simulink library "lib_energy_storage2"  (Simulink 4.1.1)
values from neighbouring files (symbols this model uses):
  logFlag = 1    [advSACompMaskInit.m]    (also in advSACompMaskInitR13.m)
undefined symbols (not defined in the file or in its folder): air_cp, amb_tmp, cyc_mph, enable_stop, ess_cap_scale, ess_cb, ess_cc, ess_coulombic_eff, ess_init_soc, ess_max_ah_cap, ess_max_p, ess_max_p_soc, ess_max_soc, ess_max_volts, ess_min_soc, ess_min_volts, ess_MMi, ess_MMo, ess_mod_airflow, ess_mod_cp, ess_mod_cpm, ess_mod_init_tmp, ess_module_mass, ess_module_num, ess_on, ess_parallel_mod_num, ess_res_scale_coef, ess_res_scale_fun, ess_set_tmp, ess_soc, ess_th_calc, ess_th_res, ess_th_res_off, ess_th_res_on, ess_tmp, ess_voc, fund_byu, fund_byuop, mc_min_volts, saber_air_temp, Saber_Battery_IO_File, saber_init_soc, saber_init_temp, saber_init_voc, saber_k_cb, saber_k_cc, saber_k_rc, saber_k_re, saber_k_rt, saber_k_soc, t_soc, time_step
libraries: simulink3 x16, lib_energy_storage x1, lib_energy_storage2 x1
(part 9 of 10)

== system lib_energy_storage2/energy storage <ess> Saber/energy storage <ess> Saber/model/Voltages ==
  Saber Voltages : Inport  Port=1  LatchInput=off
  # batteries : Gain  Gain=ess_module_num  Multiplication=Element-wise(K.*u)  SaturateOnIntegerOverflow=on
  Sum : Sum  Inputs=1  SaturateOnIntegerOverflow=on
  enhancedToWorkspace : Subsystem  TreatAsAtomicUnit=on  mask(enhancedToWorkspace){generalName=generalName, specificName=saber_ess_voltage, logFlag=logFlag}
      mask prompts: generalName "General Name [char-evaluated]"; specificName "Specific Name [char-literal]"; logFlag "Enable flag (1=on,0=off)"
      mask help: A wrapper for the Simulink "To Workspace" block that allows you to evaluate the name of the variable to log to workspace. This is useful to avoid the double logging errors that occur when you pull in two library models that attempt to log to the same variable.
      mask init:
      | enhancedToWsMaker
      settings: CopyFcn=breakLinkCopyFcn  ParentCloseFcn=breakLinkParCloseFcn  RTWFcnNameOpts=Auto  RTWFileNameOpts=Auto
      mask Help:
      | <h2>Enhanced To Workspace Block</h2>
      | <h3>Parameters</h3>
      | <UL>
      | <li><b>General Name:</b> This is the more general name of the variable. Variables are saved to the workspace as <i>generalName_specificName</i>. Note that this is an evaluated variable. If you would like to type in the value directly, it must be surrounded with single quotes. Otherwise you can input the name of a variable containing a char string.</li>
      | <li><b>Specific Name:</b> This is the specific name of the variable. Note that this is input as a char literal (i.e., you don't need quotes).</li>
      | <li><b>Enable Flag:</b> This flag should have the value of 0 or 1. If 0, the variable will not be logged to the workspace. If 1, the variable will be logged. This is done so that variable logging can be turned off to improve speed.</li>
      | </ul>
      | <h3>Overview</h3>
      | <p>The enhanced to workspace block was put together to allow one to dynamically resolve variable names at run time in simulink. This is most powerful when used in conjunction with a masked subsystem to allow multiple instances of that masked subsytem to be used in the same model. The strategy is to set the generalName in the block mask which will allow the block to change the general name for all variable logging on the fly.
      | <h3>Helper Files</h3>
      | <p>Three m-files are required by the enhancedToWorkspace block. These files are located in the &lt; ADVISOR root &gt;/GUI directory :
      | <ul>
      | <li><i>enhancedToWsMaker.m</i> This file runs the mask initialization for the block</li>
      | <li><i>breakLinkCopyFcn.m</i> This file is used by the block callback when the simulink block is copied. It is necessary to break the link to the enhancedToWorkspace similar to the To Workspace block in order for it to be able to configure itself. (Try copying simulink's To Workspace block--it is impossible to make a link)</li>
      | <li><i>breakLinkParCloseFcn.m</i> This file is similar to the breakLinkCopyFcn and is used when a parent system is closed</li>
      | </ul>
      | <hr>
      | 
      | <p>Created 2003-Jan-21, Michael Patrick O'Keefe, NREL</p>
      | 
      | <!--
      | <VARDEF>
      | <H3>var_name</H3>
      | <UL>
      | <LI><B>data type</B> data type here</LI>
      | <LI><B>units</B> units here</LI>
      | <LI><B>vehicle type</B> vehicle type here</LI>
      | <LI><B>description</B> description here</LI>
      | </UL>
      | </VARDEF>
      | -->
      mask Display: disp([generalName,'_',specificName])
  enhancedToWorkspace1 : Subsystem  TreatAsAtomicUnit=on  mask(enhancedToWorkspace){generalName=generalName, specificName=voltage, logFlag=logFlag}
      mask prompts: generalName "General Name [char-evaluated]"; specificName "Specific Name [char-literal]"; logFlag "Enable flag (1=on,0=off)"
      mask help: A wrapper for the Simulink "To Workspace" block that allows you to evaluate the name of the variable to log to workspace. This is useful to avoid the double logging errors that occur when you pull in two library models that attempt to log to the same variable.
      mask init:
      | enhancedToWsMaker
      settings: CopyFcn=breakLinkCopyFcn  ParentCloseFcn=breakLinkParCloseFcn  RTWFcnNameOpts=Auto  RTWFileNameOpts=Auto
      mask Help:
      | <h2>Enhanced To Workspace Block</h2>
      | <h3>Parameters</h3>
      | <UL>
      | <li><b>General Name:</b> This is the more general name of the variable. Variables are saved to the workspace as <i>generalName_specificName</i>. Note that this is an evaluated variable. If you would like to type in the value directly, it must be surrounded with single quotes. Otherwise you can input the name of a variable containing a char string.</li>
      | <li><b>Specific Name:</b> This is the specific name of the variable. Note that this is input as a char literal (i.e., you don't need quotes).</li>
      | <li><b>Enable Flag:</b> This flag should have the value of 0 or 1. If 0, the variable will not be logged to the workspace. If 1, the variable will be logged. This is done so that variable logging can be turned off to improve speed.</li>
      | </ul>
      | <h3>Overview</h3>
      | <p>The enhanced to workspace block was put together to allow one to dynamically resolve variable names at run time in simulink. This is most powerful when used in conjunction with a masked subsystem to allow multiple instances of that masked subsytem to be used in the same model. The strategy is to set the generalName in the block mask which will allow the block to change the general name for all variable logging on the fly.
      | <h3>Helper Files</h3>
      | <p>Three m-files are required by the enhancedToWorkspace block. These files are located in the &lt; ADVISOR root &gt;/GUI directory :
      | <ul>
      | <li><i>enhancedToWsMaker.m</i> This file runs the mask initialization for the block</li>
      | <li><i>breakLinkCopyFcn.m</i> This file is used by the block callback when the simulink block is copied. It is necessary to break the link to the enhancedToWorkspace similar to the To Workspace block in order for it to be able to configure itself. (Try copying simulink's To Workspace block--it is impossible to make a link)</li>
      | <li><i>breakLinkParCloseFcn.m</i> This file is similar to the breakLinkCopyFcn and is used when a parent system is closed</li>
      | </ul>
      | <hr>
      | 
      | <p>Created 2003-Jan-21, Michael Patrick O'Keefe, NREL</p>
      | 
      | <!--
      | <VARDEF>
      | <H3>var_name</H3>
      | <UL>
      | <LI><B>data type</B> data type here</LI>
      | <LI><B>units</B> units here</LI>
      | <LI><B>vehicle type</B> vehicle type here</LI>
      | <LI><B>description</B> description here</LI>
      | </UL>
      | </VARDEF>
      | -->
      mask Display: disp([generalName,'_',specificName])
  ADV Voltage : Outport  Port=1
  tag scope: bus_voltage=scoped
  wires:
  # batteries/1 -> Sum/1, enhancedToWorkspace/1(In1)
  Sum/1 -> [bus_voltage], enhancedToWorkspace1/1(In1), ADV Voltage/1
  Saber Voltages/1 -> # batteries/1

== system lib_energy_storage2/energy storage <ess> Saber/energy storage <ess> Saber/model/enhancedToWorkspace ==
  In1 : Inport  Port=1  LatchInput=off
  Terminator : Terminator
  wires:
  In1/1 -> Terminator/1

== system lib_energy_storage2/energy storage <ess> Saber/energy storage <ess> Saber/model/max pack pwr (W) ==
  note: Edit in the future
      | Used in series power follower
  Ground : Ground
  tag scope: ess_max_pwr=scoped
  wires:
  Ground/1 -> [ess_max_pwr]

== system lib_energy_storage2/energy storage <ess> fundamental model/energy storage <ess> fundamental model/model/Block NOTES ==
  note: Fundamentally based SOC model developed at BYU
      | Files needed:
      | input1.dat
      | input2.dat
      | input3.dat
      | nrel13cs.dll

== system lib_energy_storage2/energy storage <ess> fundamental model/energy storage <ess> fundamental model/model/enhancedToWorkspace ==
  In1 : Inport  Port=1  LatchInput=off
  Terminator : Terminator
  wires:
  In1/1 -> Terminator/1

== system lib_energy_storage2/energy storage <ess> fundamental model/energy storage <ess> fundamental model/model/enhancedToWorkspace1 ==
  In1 : Inport  Port=1  LatchInput=off
  Terminator : Terminator
  wires:
  In1/1 -> Terminator/1

== system lib_energy_storage2/energy storage <ess> fundamental model/energy storage <ess> fundamental model/model/enhancedToWorkspace2 ==
  In1 : Inport  Port=1  LatchInput=off
  Terminator : Terminator
  wires:
  In1/1 -> Terminator/1

== system lib_energy_storage2/energy storage <ess> fundamental model/energy storage <ess> fundamental model/model/enhancedToWorkspace3 ==
  In1 : Inport  Port=1  LatchInput=off
  Terminator : Terminator
  wires:
  In1/1 -> Terminator/1

== system lib_energy_storage2/energy storage <ess> fundamental model/energy storage <ess> fundamental model/model/enhancedToWorkspace4 ==
  In1 : Inport  Port=1  LatchInput=off
  Terminator : Terminator
  wires:
  In1/1 -> Terminator/1

== system lib_energy_storage2/energy storage <ess> fundamental model/energy storage <ess> fundamental model/model/enhancedToWorkspace5 ==
  In1 : Inport  Port=1  LatchInput=off
  Terminator : Terminator
  wires:
  In1/1 -> Terminator/1

== system lib_energy_storage2/energy storage <ess> fundamental model/energy storage <ess> fundamental model/model/enhancedToWorkspace6 ==
  In1 : Inport  Port=1  LatchInput=off
  Terminator : Terminator
  wires:
  In1/1 -> Terminator/1

== system lib_energy_storage2/energy storage <ess> fundamental model/energy storage <ess> fundamental model/model/enhancedToWorkspace7 ==
  In1 : Inport  Port=1  LatchInput=off
  Terminator : Terminator
  wires:
  In1/1 -> Terminator/1

== system lib_energy_storage2/energy storage <ess> fundamental model/energy storage <ess> fundamental model/model/ess tmp ==
  Qess_gen : Inport  Port=1  LatchInput=off
  Enable : EnablePort  StatesWhenEnabling=reset
  #of mods : Gain  Gain=ess_module_num  Multiplication=Element-wise(K.*u)  SaturateOnIntegerOverflow=on
  1/#of mods : Gain  Gain=1/ess_module_num  Multiplication=Element-wise(K.*u)  SaturateOnIntegerOverflow=on
  1/mcp : Gain  Gain=1/(ess_module_mass*ess_mod_cp)  Multiplication=Element-wise(K.*u)  SaturateOnIntegerOverflow=on
  Block NOTES : Subsystem
      settings: RTWFcnNameOpts=Auto  RTWFileNameOpts=Auto
      mask Display: disp('Block\nNOTES')
  Memory : Memory  Orientation=left  X0=cyc_mph(1,2)*.447  InheritSampleTime=off
      settings: RTWStateStorageClass=Auto
  Memory1 : Memory  Orientation=left  X0=cyc_mph(1,2)*.447  InheritSampleTime=off
      settings: RTWStateStorageClass=Auto
  Mux20 : Mux  Inputs=3
      settings: DisplayOption=none
  Qc : Sum  Inputs=++  SaturateOnIntegerOverflow=on
  Qess_case : Fcn  Expr=(u(2) - u(1))/u(3)
  Saturation3 : Saturate  Orientation=left  UpperLimit=1  LowerLimit=0  LinearizeAsGain=on
  Tair,ave : Subsystem  TreatAsAtomicUnit=on
      settings: RTWFcnNameOpts=Auto  RTWFileNameOpts=Auto
  Tess2 : Integrator  ExternalReset=none  InitialConditionSource=internal  InitialCondition=ess_mod_init_tmp  LimitOutput=off  UpperSaturationLimit=inf  LowerSaturationLimit=-inf  ShowSaturationPort=off  ShowStatePort=off  AbsoluteTolerance=auto
  thermostat : Fcn  Orientation=left  Expr=u(1) - ess_set_tmp
  Tess : Outport  Port=1  InitialOutput=0
  Tair : Outport  Port=2
  Qair : Outport  Port=3  OutputWhenDisabled=reset  InitialOutput=0
  wires:
  Tair,ave/1(Tair_ave) -> Tair/1, Mux20/2
  Tair,ave/2(Th Res) -> Mux20/3
  Mux20/1 -> Qess_case/1
  #of mods/1 -> Qair/1
  Memory/1 -> Tair,ave/1(Qess_case)
  Memory1/1 -> Tair,ave/Enable
  Saturation3/1 -> Memory1/1
  thermostat/1 -> Saturation3/1
  1/#of mods/1 -> Qc/2
  Qess_gen/1 -> 1/#of mods/1
  Tess2/1 -> thermostat/1, Mux20/1, Tess/1
  1/mcp/1 -> Tess2/1
  Qess_case/1 -> #of mods/1, Memory/1, Qc/1
  Qc/1 -> 1/mcp/1

== system lib_energy_storage2/energy storage <ess> fundamental model/energy storage <ess> fundamental model/model/max pack pwr (W) ==
  SOC : Inport  Port=1  LatchInput=off
  # batteries : Gain  Gain=ess_module_num  Multiplication=Element-wise(K.*u)  SaturateOnIntegerOverflow=on
  max power : Lookup  InputValues=ess_max_p_soc  OutputValues=ess_max_p
  ess discharge pwr : Outport  Port=1  InitialOutput=0
  wires:
  # batteries/1 -> ess discharge pwr/1
  max power/1 -> # batteries/1
  SOC/1 -> max power/1

== system lib_energy_storage2/energy storage <ess> fundamental model/energy storage <ess> fundamental model/model/stop sim ==
  SOC : Inport  Port=1  LatchInput=off
  Enable : EnablePort
  Const : Constant  Orientation=up  Value=0.1
  Relational Operator : RelationalOperator  Operator=<
  Stop Simulation : Stop
  wires:
  Relational Operator/1 -> Stop Simulation/1
  SOC/1 -> Relational Operator/1
  Const/1 -> Relational Operator/2

== system lib_energy_storage2/energy storage <ess> optima fundamental model/energy storage <ess> optima fundamental model/model/Block NOTES ==
  note: Fundamentally based SOC model developed at BYU
      | Files needed:
      | input1.dat
      | input2.dat
      | input3.dat
      | nrel13cs.dll

== system lib_energy_storage2/energy storage <ess> optima fundamental model/energy storage <ess> optima fundamental model/model/enhancedToWorkspace ==
  In1 : Inport  Port=1  LatchInput=off
  Terminator : Terminator
  wires:
  In1/1 -> Terminator/1

== system lib_energy_storage2/energy storage <ess> optima fundamental model/energy storage <ess> optima fundamental model/model/enhancedToWorkspace1 ==
  In1 : Inport  Port=1  LatchInput=off
  Terminator : Terminator
  wires:
  In1/1 -> Terminator/1

== system lib_energy_storage2/energy storage <ess> optima fundamental model/energy storage <ess> optima fundamental model/model/enhancedToWorkspace2 ==
  In1 : Inport  Port=1  LatchInput=off
  Terminator : Terminator
  wires:
  In1/1 -> Terminator/1

== system lib_energy_storage2/energy storage <ess> optima fundamental model/energy storage <ess> optima fundamental model/model/enhancedToWorkspace3 ==
  In1 : Inport  Port=1  LatchInput=off
  Terminator : Terminator
  wires:
  In1/1 -> Terminator/1

== system lib_energy_storage2/energy storage <ess> optima fundamental model/energy storage <ess> optima fundamental model/model/enhancedToWorkspace4 ==
  In1 : Inport  Port=1  LatchInput=off
  Terminator : Terminator
  wires:
  In1/1 -> Terminator/1

== system lib_energy_storage2/energy storage <ess> optima fundamental model/energy storage <ess> optima fundamental model/model/enhancedToWorkspace5 ==
  In1 : Inport  Port=1  LatchInput=off
  Terminator : Terminator
  wires:
  In1/1 -> Terminator/1

== system lib_energy_storage2/energy storage <ess> optima fundamental model/energy storage <ess> optima fundamental model/model/enhancedToWorkspace6 ==
  In1 : Inport  Port=1  LatchInput=off
  Terminator : Terminator
  wires:
  In1/1 -> Terminator/1

== system lib_energy_storage2/energy storage <ess> optima fundamental model/energy storage <ess> optima fundamental model/model/enhancedToWorkspace7 ==
  In1 : Inport  Port=1  LatchInput=off
  Terminator : Terminator
  wires:
  In1/1 -> Terminator/1

== system lib_energy_storage2/energy storage <ess> optima fundamental model/energy storage <ess> optima fundamental model/model/ess tmp ==
  Qess_gen : Inport  Port=1  LatchInput=off
  Enable : EnablePort  StatesWhenEnabling=reset
  #of mods : Gain  Gain=ess_module_num  Multiplication=Element-wise(K.*u)  SaturateOnIntegerOverflow=on
  1/#of mods : Gain  Gain=1/ess_module_num  Multiplication=Element-wise(K.*u)  SaturateOnIntegerOverflow=on
  1/mcp : Gain  Gain=1/(ess_module_mass*ess_mod_cp)  Multiplication=Element-wise(K.*u)  SaturateOnIntegerOverflow=on
  Block NOTES : Subsystem
      settings: RTWFcnNameOpts=Auto  RTWFileNameOpts=Auto
      mask Display: disp('Block\nNOTES')
  Memory : Memory  Orientation=left  X0=cyc_mph(1,2)*.447  InheritSampleTime=off
      settings: RTWStateStorageClass=Auto
  Memory1 : Memory  Orientation=left  X0=cyc_mph(1,2)*.447  InheritSampleTime=off
      settings: RTWStateStorageClass=Auto
  Mux20 : Mux  Inputs=3
      settings: DisplayOption=none
  Qc : Sum  Inputs=++  SaturateOnIntegerOverflow=on
  Qess_case : Fcn  Expr=(u(2) - u(1))/u(3)
  Saturation3 : Saturate  Orientation=left  UpperLimit=1  LowerLimit=0  LinearizeAsGain=on
  Tair,ave : Subsystem  TreatAsAtomicUnit=on
      settings: RTWFcnNameOpts=Auto  RTWFileNameOpts=Auto
  Tess2 : Integrator  ExternalReset=none  InitialConditionSource=internal  InitialCondition=ess_mod_init_tmp  LimitOutput=off  UpperSaturationLimit=inf  LowerSaturationLimit=-inf  ShowSaturationPort=off  ShowStatePort=off  AbsoluteTolerance=auto
  thermostat : Fcn  Orientation=left  Expr=u(1) - ess_set_tmp
  Tess : Outport  Port=1  InitialOutput=0
  Tair : Outport  Port=2
  Qair : Outport  Port=3  OutputWhenDisabled=reset  InitialOutput=0
  wires:
  Tair,ave/1(Tair_ave) -> Tair/1, Mux20/2
  Tair,ave/2(Th Res) -> Mux20/3
  Mux20/1 -> Qess_case/1
  #of mods/1 -> Qair/1
  Memory/1 -> Tair,ave/1(Qess_case)
  Memory1/1 -> Tair,ave/Enable
  Saturation3/1 -> Memory1/1
  thermostat/1 -> Saturation3/1
  1/#of mods/1 -> Qc/2
  Qess_gen/1 -> 1/#of mods/1
  Tess2/1 -> thermostat/1, Mux20/1, Tess/1
  1/mcp/1 -> Tess2/1
  Qess_case/1 -> #of mods/1, Memory/1, Qc/1
  Qc/1 -> 1/mcp/1

== system lib_energy_storage2/energy storage <ess> optima fundamental model/energy storage <ess> optima fundamental model/model/max pack pwr (W) ==
  SOC : Inport  Port=1  LatchInput=off
  # batteries : Gain  Gain=ess_module_num  Multiplication=Element-wise(K.*u)  SaturateOnIntegerOverflow=on
  max power : Lookup  InputValues=ess_max_p_soc  OutputValues=ess_max_p
  ess discharge pwr : Outport  Port=1  InitialOutput=0
  wires:
  # batteries/1 -> ess discharge pwr/1
  max power/1 -> # batteries/1
  SOC/1 -> max power/1

== system lib_energy_storage2/energy storage <ess> optima fundamental model/energy storage <ess> optima fundamental model/model/stop sim ==
  SOC : Inport  Port=1  LatchInput=off
  Enable : EnablePort
  Const : Constant  Orientation=up  Value=.001
  Relational Operator : RelationalOperator  Operator=<
  Stop Simulation : Stop
  wires:
  Relational Operator/1 -> Stop Simulation/1
  SOC/1 -> Relational Operator/1
  Const/1 -> Relational Operator/2

== system lib_energy_storage2/Ultracapacitor  System/Ultracapacitor  System/model/Calc Iout/SOC limit ==
  SOC : Inport  Port=1  LatchInput=off
  Pbty : Inport  Port=2  LatchInput=off
  Constant1 : Constant  Value=0.001
  Constant5 : Constant  Value=.999
  Constant9 : Constant  Value=0
  Logical Operator : Logic  Operator=OR  Inputs=2
  Logical Operator1 : Logic  Operator=AND  Inputs=2
  Logical Operator2 : Logic  Operator=NOT  Inputs=1
  Relational Operator : RelationalOperator  Operator=>
  Relational Operator3 : RelationalOperator  Operator=<
  SOC>=.999 : RelationalOperator  Operator=>=
  charging (Preq is neg) : RelationalOperator  Operator=<
  no power req if SOC<0 and trying  to discharge : Switch  Threshold=eps
  no power req if SOC>.999 and trying  to charge : Switch  Threshold=eps
  "Pbty, limited" : Outport  Port=1  InitialOutput=0
  tag scope: ess_soc_hi_limited=scoped, ess_soc_low_limited=scoped
  wires:
  Constant1/1 -> Relational Operator/2
  Pbty/1 -> Relational Operator3/1, charging (Preq is neg)/1, no power req if SOC<0 and trying  to discharge/1
  Logical Operator/1 -> Logical Operator2/1, no power req if SOC<0 and trying  to discharge/2
  SOC/1 -> Relational Operator/1, SOC>=.999/1
  SOC>=.999/1 -> Logical Operator1/1
  charging (Preq is neg)/1 -> Logical Operator1/2
  Constant5/1 -> SOC>=.999/2
  no power req if SOC<0 and trying  to discharge/1 -> no power req if SOC>.999 and trying  to charge/3
  no power req if SOC>.999 and trying  to charge/1 -> "Pbty, limited"/1
  Logical Operator1/1 -> [ess_soc_hi_limited], no power req if SOC>.999 and trying  to charge/2
  Relational Operator3/1 -> Logical Operator/2
  Constant9/1 -> Relational Operator3/2, charging (Preq is neg)/2, no power req if SOC<0 and trying  to discharge/3, no power req if SOC>.999 and trying  to charge/1
  Relational Operator/1 -> Logical Operator/1
  Logical Operator2/1 -> [ess_soc_low_limited]

== system lib_energy_storage2/Ultracapacitor  System/Ultracapacitor  System/model/Calc Iout/enhancedToWorkspace ==
  In1 : Inport  Port=1  LatchInput=off
  Terminator : Terminator
  wires:
  In1/1 -> Terminator/1

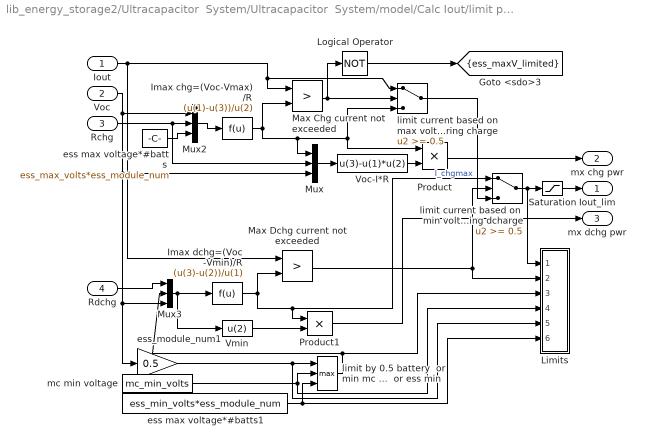
== system lib_energy_storage2/Ultracapacitor  System/Ultracapacitor  System/model/Calc Iout/limit power ==
  Iout : Inport  Port=1  LatchInput=off
  Voc : Inport  Port=2  LatchInput=off
  Rchg : Inport  Port=3  LatchInput=off
  Rdchg : Inport  Port=4  LatchInput=off
  Imax chg=(Voc-Vmax)/R : Fcn  Expr=(u(1)-u(3))/u(2)
  Imax dchg=(Voc -Vmin)/R : Fcn  Expr=(u(3)-u(2))/u(1)
  Limits : Subsystem
      settings: RTWFcnNameOpts=Auto  RTWFileNameOpts=Auto
  Logical Operator : Logic  Operator=NOT  Inputs=2
  Max Chg current not exceeded : RelationalOperator  Operator=>
  Max Dchg current not exceeded : RelationalOperator  Operator=>
  Mux : Mux  Inputs=3
  Mux2 : Mux  Inputs=3
  Mux3 : Mux  Inputs=3
  Product : Product  Inputs=2  Multiplication=Element-wise(.*)  SaturateOnIntegerOverflow=on
  Product1 : Product  Inputs=2  Multiplication=Element-wise(.*)  SaturateOnIntegerOverflow=on
  Saturation : Saturate  UpperLimit=2000*ess_parallel_mod_num  LowerLimit=-2000*ess_parallel_mod_num  LinearizeAsGain=on
  Vmin : Fcn  Expr=u(2)
  Voc-I*R : Fcn  Expr=u(3)-u(1)*u(2)
  ess max voltage*#batts : Constant  Value=ess_max_volts*ess_module_num
  ess max voltage*#batts1 : Constant  Value=ess_min_volts*ess_module_num
  ess_module_num1 : Gain  Gain=0.5  Multiplication=Element-wise(K.*u)  SaturateOnIntegerOverflow=on
  limit by 0.5 battery  or min mc voltage  or ess min : MinMax  Function=max  Inputs=3
  limit current based on  max voltage during charge : Switch  Threshold=0.5
  limit current based on  min voltage during dcharge : Switch  Threshold=0.5
  mc min voltage : Constant  Value=mc_min_volts
  Iout_lim : Outport  Port=1
  mx chg pwr : Outport  Port=2
  mx dchg pwr : Outport  Port=3
  tag scope: ess_maxV_limited=scoped
  wires:
  Mux2/1 -> Imax chg=(Voc-Vmax)/R/1
  Iout/1 -> Max Chg current not exceeded/1, limit current based on  max voltage during charge/1, Max Dchg current not exceeded/1
  Imax chg=(Voc-Vmax)/R/1 -> Max Chg current not exceeded/2, Mux/1, limit current based on  max voltage during charge/3, Product/1
  Rchg/1 -> Mux2/2, Mux/2
  Voc/1 -> Mux2/1, Mux/3, Mux3/3, ess_module_num1/1
  Mux/1 -> Voc-I*R/1
  Voc-I*R/1 -> Product/2
  Product/1 -> mx chg pwr/1
  Max Chg current not exceeded/1 -> limit current based on  max voltage during charge/2, Logical Operator/1
  Logical Operator/1 -> [ess_maxV_limited]
  ess max voltage*#batts/1 -> Mux2/3
  limit current based on  max voltage during charge/1 -> limit current based on  min voltage during dcharge/3  "I_chgmax"
  limit current based on  min voltage during dcharge/1 -> Saturation/1, Limits/1(current req)
  Mux3/1 -> Imax dchg=(Voc -Vmin)/R/1, Vmin/1
  Imax dchg=(Voc -Vmin)/R/1 -> Max Dchg current not exceeded/2, Product1/1, limit current based on  min voltage during dcharge/1
  ess max voltage*#batts1/1 -> limit by 0.5 battery  or min mc voltage  or ess min/3, Limits/6(V ess_min_volts)
  Rdchg/1 -> Mux3/1
  Max Dchg current not exceeded/1 -> limit current based on  min voltage during dcharge/2, Limits/2(current bat limited)
  mc min voltage/1 -> limit by 0.5 battery  or min mc voltage  or ess min/2, Limits/4(V mc_min_volts)
  ess_module_num1/1 -> limit by 0.5 battery  or min mc voltage  or ess min/1, Limits/5(V battery (.5Voc))
  limit by 0.5 battery  or min mc voltage  or ess min/1 -> Limits/3(V used), Mux3/2
  Vmin/1 -> Product1/2
  Product1/1 -> mx dchg pwr/1
  Saturation/1 -> Iout_lim/1

== system lib_energy_storage2/Ultracapacitor  System/Ultracapacitor  System/model/ess tmp/Block NOTES ==
  note: This block models the thermal behavior of a battery module with active air cooling.
      | The module is modeled as a single lumped thermal mass.
      | The fan is on whenever the battery temp is > the set temp.

== system lib_energy_storage2/Ultracapacitor  System/Ultracapacitor  System/model/ess tmp/Tair,ave ==
  Qess_case : Inport  Port=1  LatchInput=off
  Enable : EnablePort  StatesWhenEnabling=reset
  Block NOTES : Subsystem
      settings: RTWFcnNameOpts=Auto  RTWFileNameOpts=Auto
      mask Display: disp('Block\nNOTES')
  Tamb-(Q/mcp)/2 : Fcn  Expr=amb_tmp - (u(1)/(ess_mod_airflow*air_cp))/2
  do ex calcs?1 : Constant  Value=ess_th_res_on
  Tair_ave : Outport  Port=1  OutputWhenDisabled=reset  InitialOutput=amb_tmp
  Th Res : Outport  Port=2  OutputWhenDisabled=reset  InitialOutput=ess_th_res_off
  wires:
  Tamb-(Q/mcp)/2/1 -> Tair_ave/1
  Qess_case/1 -> Tamb-(Q/mcp)/2/1
  do ex calcs?1/1 -> Th Res/1

== system lib_energy_storage2/energy storage <ess>/energy storage <ess>/Model/compute current/enhancedToWorkspace2 ==
  In1 : Inport  Port=1  LatchInput=off
  Terminator : Terminator
  wires:
  In1/1 -> Terminator/1

== system lib_energy_storage2/energy storage <ess>/energy storage <ess>/Model/ess tmp/Block NOTES ==
  note: This block models the thermal behavior of a battery module with active air cooling.
      | The module is modeled as a single lumped thermal mass.
      | The fan is on whenever the battery temp is > the set temp.

== system lib_energy_storage2/energy storage <ess>/energy storage <ess>/Model/ess tmp/Tair,ave ==
  Qess_case : Inport  Port=1  LatchInput=off
  Enable : EnablePort  StatesWhenEnabling=reset
  Block NOTES : Subsystem
      settings: RTWFcnNameOpts=Auto  RTWFileNameOpts=Auto
      mask Display: disp('Block\nNOTES')
  Tamb-(Q/mcp)/2 : Fcn  Expr=amb_tmp - (u(1)/(ess_mod_airflow*air_cp))/2
  do ex calcs?1 : Constant  Value=ess_th_res_on
  Tair_ave : Outport  Port=1  OutputWhenDisabled=reset  InitialOutput=amb_tmp
  Th Res : Outport  Port=2  OutputWhenDisabled=reset  InitialOutput=ess_th_res_off
  wires:
  do ex calcs?1/1 -> Th Res/1
  Qess_case/1 -> Tamb-(Q/mcp)/2/1
  Tamb-(Q/mcp)/2/1 -> Tair_ave/1

== system lib_energy_storage2/energy storage <ess>/energy storage <ess>/Model/limit power/Limits ==
  SOC  high limited : Inport  Port=1  LatchInput=off
  not SOC  low limited : Inport  Port=2  LatchInput=off
  power req : Inport  Port=3  LatchInput=off
  power bat limited : Inport  Port=4  LatchInput=off
  V used : Inport  Port=5  LatchInput=off
  V mc_min_volts : Inport  Port=6  LatchInput=off
  V battery (.5Voc) : Inport  Port=7  LatchInput=off
  V ess_min_volts : Inport  Port=8  LatchInput=off
  Logical Operator1 : Logic  Operator=NOT  Inputs=1
  Relational Operator{1,3..5} (4 alike) : RelationalOperator  Operator===
  limited by battery : Logic  Operator=AND  Inputs=2
  limited by battery min V : Logic  Operator=AND  Inputs=2
  limited by motor controller : Logic  Operator=AND  Inputs=2
  tag scope: ess_minV_limited=scoped, ess_pwr_limited=scoped, ess_soc_hi_limited=scoped, ess_soc_low_limited=scoped, mc_voltage_limited=scoped
  wires:
  SOC  high limited/1 -> [ess_soc_hi_limited]
  not SOC  low limited/1 -> Logical Operator1/1
  Logical Operator1/1 -> [ess_soc_low_limited]
  power req/1 -> Relational Operator1/1
  Relational Operator5/1 -> limited by battery min V/2
  Relational Operator4/1 -> limited by battery/2
  Relational Operator1/1 -> limited by battery min V/1, limited by battery/1, limited by motor controller/1
  Relational Operator3/1 -> limited by motor controller/2
  limited by battery min V/1 -> [ess_minV_limited]
  limited by battery/1 -> [ess_pwr_limited]
  limited by motor controller/1 -> [mc_voltage_limited]
  V ess_min_volts/1 -> Relational Operator5/2
  V battery (.5Voc)/1 -> Relational Operator4/2
  V used/1 -> Relational Operator5/1, Relational Operator4/1, Relational Operator3/1
  V mc_min_volts/1 -> Relational Operator3/2
  power bat limited/1 -> Relational Operator1/2

== system lib_energy_storage2/energy storage <ess>/energy storage <ess>/Model/max pack pwr (W)1/Rchg (ohms)1 ==
  x0 : Inport  Port=1  LatchInput=off
  y0 : Inport  Port=2  LatchInput=off
  Mux : Mux  Inputs=2
      settings: DisplayOption=none
  S-function : S-Function  FunctionName=sftable2  Parameters=xindex, yindex, table  PortCounts=[]  SFunctionModules=''
  table out : Outport  Port=1  InitialOutput=0
  wires:
  y0/1 -> Mux/2
  S-function/1 -> table out/1
  x0/1 -> Mux/1
  Mux/1 -> S-function/1

== system lib_energy_storage2/energy storage <ess>/energy storage <ess>/Model/max pack pwr (W)1/Rdis (ohms) ==
  x0 : Inport  Port=1  LatchInput=off
  y0 : Inport  Port=2  LatchInput=off
  Mux : Mux  Inputs=2
      settings: DisplayOption=none
  S-function : S-Function  FunctionName=sftable2  Parameters=xindex, yindex, table  PortCounts=[]  SFunctionModules=''
  table out : Outport  Port=1  InitialOutput=0
  wires:
  y0/1 -> Mux/2
  S-function/1 -> table out/1
  x0/1 -> Mux/1
  Mux/1 -> S-function/1

== system lib_energy_storage2/energy storage <ess>/energy storage <ess>/Model/max pack pwr (W)1/VOC (V) ==
  x0 : Inport  Port=1  LatchInput=off
  y0 : Inport  Port=2  LatchInput=off
  Mux : Mux  Inputs=2
      settings: DisplayOption=none
  S-function : S-Function  FunctionName=sftable2  Parameters=xindex, yindex, table  PortCounts=[]  SFunctionModules=''
  table out : Outport  Port=1  InitialOutput=0
  wires:
  y0/1 -> Mux/2
  S-function/1 -> table out/1
  x0/1 -> Mux/1
  Mux/1 -> S-function/1

== system lib_energy_storage2/energy storage <ess>/energy storage <ess>/Model/pack Voc, Rint/Rchg (ohms) ==
  x0 : Inport  Port=1  LatchInput=off
  y0 : Inport  Port=2  LatchInput=off
  Mux : Mux  Inputs=2
      settings: DisplayOption=none
  S-function : S-Function  FunctionName=sftable2  Parameters=xindex, yindex, table  PortCounts=[]  SFunctionModules=''
  table out : Outport  Port=1  InitialOutput=0
  wires:
  Mux/1 -> S-function/1
  x0/1 -> Mux/1
  S-function/1 -> table out/1
  y0/1 -> Mux/2

== system lib_energy_storage2/energy storage <ess>/energy storage <ess>/Model/pack Voc, Rint/Rdis (ohms) ==
  x0 : Inport  Port=1  LatchInput=off
  y0 : Inport  Port=2  LatchInput=off
  Mux : Mux  Inputs=2
      settings: DisplayOption=none
  S-function : S-Function  FunctionName=sftable2  Parameters=xindex, yindex, table  PortCounts=[]  SFunctionModules=''
  table out : Outport  Port=1  InitialOutput=0
  wires:
  Mux/1 -> S-function/1
  x0/1 -> Mux/1
  S-function/1 -> table out/1
  y0/1 -> Mux/2

== system lib_energy_storage2/energy storage <ess>/energy storage <ess>/Model/pack Voc, Rint/VOC (V) ==
  x0 : Inport  Port=1  LatchInput=off
  y0 : Inport  Port=2  LatchInput=off
  Mux : Mux  Inputs=2
      settings: DisplayOption=none
  S-function : S-Function  FunctionName=sftable2  Parameters=xindex, yindex, table  PortCounts=[]  SFunctionModules=''
  table out : Outport  Port=1  InitialOutput=0
  wires:
  Mux/1 -> S-function/1
  x0/1 -> Mux/1
  S-function/1 -> table out/1
  y0/1 -> Mux/2

== system lib_energy_storage2/energy storage <ess> RC/energy storage <ess> RC/model/Model Parameters/rc ==
  x0 : Inport  Port=1  LatchInput=off
  y0 : Inport  Port=2  LatchInput=off
  Mux : Mux  Inputs=2
      settings: DisplayOption=none
  S-function : S-Function  FunctionName=sftable2  Parameters=xindex, yindex, table  PortCounts=[]  SFunctionModules=''
  table out : Outport  Port=1  InitialOutput=0
  wires:
  y0/1 -> Mux/2
  S-function/1 -> table out/1
  x0/1 -> Mux/1
  Mux/1 -> S-function/1

== system lib_energy_storage2/energy storage <ess> RC/energy storage <ess> RC/model/Model Parameters/re ==
  x0 : Inport  Port=1  LatchInput=off
  y0 : Inport  Port=2  LatchInput=off
  Mux : Mux  Inputs=2
      settings: DisplayOption=none
  S-function : S-Function  FunctionName=sftable2  Parameters=xindex, yindex, table  PortCounts=[]  SFunctionModules=''
  table out : Outport  Port=1  InitialOutput=0
  wires:
  Mux/1 -> S-function/1
  x0/1 -> Mux/1
  S-function/1 -> table out/1
  y0/1 -> Mux/2

== system lib_energy_storage2/energy storage <ess> RC/energy storage <ess> RC/model/Model Parameters/rt ==
  x0 : Inport  Port=1  LatchInput=off
  y0 : Inport  Port=2  LatchInput=off
  Mux : Mux  Inputs=2
      settings: DisplayOption=none
  S-function : S-Function  FunctionName=sftable2  Parameters=xindex, yindex, table  PortCounts=[]  SFunctionModules=''
  table out : Outport  Port=1  InitialOutput=0
  wires:
  Mux/1 -> S-function/1
  x0/1 -> Mux/1
  S-function/1 -> table out/1
  y0/1 -> Mux/2

== system lib_energy_storage2/energy storage <ess> RC/energy storage <ess> RC/model/RC model/enhancedToWorkspace6 ==
  In1 : Inport  Port=1  LatchInput=off
  Terminator : Terminator
  wires:
  In1/1 -> Terminator/1

== system lib_energy_storage2/energy storage <ess> RC/energy storage <ess> RC/model/Thermal Model of Battery/Block NOTES ==
  note: This block models the thermal behavior of a battery module with active air cooling.
      | The module is modeled as a single lumped thermal mass.
      | The fan is on whenever the battery temp is > the set temp.

== system lib_energy_storage2/energy storage <ess> RC/energy storage <ess> RC/model/Thermal Model of Battery/Tair,ave ==
  Qess_case : Inport  Port=1  LatchInput=off
  Enable : EnablePort  StatesWhenEnabling=reset
  Block NOTES : Subsystem
      settings: RTWFcnNameOpts=Auto  RTWFileNameOpts=Auto
      mask Display: disp('Block\nNOTES')
  Tamb-(Q/mcp)/2 : Fcn  Expr=amb_tmp - (u(1)/(ess_mod_airflow*air_cp))/2
  do ex calcs?1 : Constant  Value=ess_th_res_on
  Tair_ave : Outport  Port=1  OutputWhenDisabled=reset  InitialOutput=amb_tmp
  Th Res : Outport  Port=2  OutputWhenDisabled=reset  InitialOutput=ess_th_res_off
  wires:
  do ex calcs?1/1 -> Th Res/1
  Qess_case/1 -> Tamb-(Q/mcp)/2/1
  Tamb-(Q/mcp)/2/1 -> Tair_ave/1

== system lib_energy_storage2/energy storage <ess> nnet/energy storage <ess> nnet/model/NNet/Neural Network ==
  "p{1}" : Inport  Port=1  LatchInput=off  PortDimensions=2
  Layer 1 : Subsystem
      settings: RTWFcnNameOpts=Auto  RTWFileNameOpts=Auto
  Layer 2 : Subsystem
      settings: RTWFcnNameOpts=Auto  RTWFileNameOpts=Auto
  "y{1}" : Outport  Port=1  InitialOutput=[0;0]
  wires:
  Layer 2/1("a{2}") -> "y{1}"/1
  [feedback1] -> Layer 2/1("a{1} ")
  Layer 1/1("a{1}") -> [feedback1]
  "p{1}"/1 -> Layer 1/1("p{1}")

== system lib_energy_storage2/energy storage <ess> nnet/energy storage <ess> nnet/model/No Thermal model/enhancedToWorkspace ==
  In1 : Inport  Port=1  LatchInput=off
  Terminator : Terminator
  wires:
  In1/1 -> Terminator/1

== system lib_energy_storage2/energy storage <ess> nnet/energy storage <ess> nnet/model/No Thermal model/enhancedToWorkspace1 ==
  In1 : Inport  Port=1  LatchInput=off
  Terminator : Terminator
  wires:
  In1/1 -> Terminator/1

== system lib_energy_storage2/energy storage <ess> nnet/energy storage <ess> nnet/model/No Thermal model/enhancedToWorkspace2 ==
  In1 : Inport  Port=1  LatchInput=off
  Terminator : Terminator
  wires:
  In1/1 -> Terminator/1

== system lib_energy_storage2/energy storage <ess> nnet/energy storage <ess> nnet/model/No Thermal model/enhancedToWorkspace3 ==
  In1 : Inport  Port=1  LatchInput=off
  Terminator : Terminator
  wires:
  In1/1 -> Terminator/1

== system lib_energy_storage2/energy storage <ess> Saber/energy storage <ess> Saber/model/Power/enhancedToWorkspace ==
  In1 : Inport  Port=1  LatchInput=off
  Terminator : Terminator
  wires:
  In1/1 -> Terminator/1

== system lib_energy_storage2/energy storage <ess> Saber/energy storage <ess> Saber/model/Power request/enhancedToWorkspace ==
  In1 : Inport  Port=1  LatchInput=off
  Terminator : Terminator
  wires:
  In1/1 -> Terminator/1

== system lib_energy_storage2/energy storage <ess> Saber/energy storage <ess> Saber/model/SOC's/Mean ==
  In : Inport  Port=1  LatchInput=off
  Average over  10 modules : Gain  Gain=1/10  Multiplication=Element-wise(K.*u)  SaturateOnIntegerOverflow=on
  Sum2 : Sum  Inputs=1  SaturateOnIntegerOverflow=on
  Out : Outport  Port=1
  wires:
  Sum2/1 -> Average over  10 modules/1
  In/1 -> Sum2/1
  Average over  10 modules/1 -> Out/1

== system lib_energy_storage2/energy storage <ess> Saber/energy storage <ess> Saber/model/SOC's/enhancedToWorkspace ==
  In1 : Inport  Port=1  LatchInput=off
  Terminator : Terminator
  wires:
  In1/1 -> Terminator/1

== system lib_energy_storage2/energy storage <ess> Saber/energy storage <ess> Saber/model/SOC's/stop sim ==
  SOC : Inport  Port=1  LatchInput=off
  Enable : EnablePort
  Const : Constant  Orientation=up  Value=0.1
  Relational Operator : RelationalOperator  Operator=<
  Stop Simulation : Stop
  wires:
  Const/1 -> Relational Operator/2
  SOC/1 -> Relational Operator/1
  Relational Operator/1 -> Stop Simulation/1

== system lib_energy_storage2/energy storage <ess> Saber/energy storage <ess> Saber/model/Temps/Mean ==
  In : Inport  Port=1  LatchInput=off
  Average over  10 modules : Gain  Gain=1/10  Multiplication=Element-wise(K.*u)  SaturateOnIntegerOverflow=on
  Sum2 : Sum  Inputs=1  SaturateOnIntegerOverflow=on
  Out : Outport  Port=1
  wires:
  Sum2/1 -> Average over  10 modules/1
  In/1 -> Sum2/1
  Average over  10 modules/1 -> Out/1

== system lib_energy_storage2/energy storage <ess> Saber/energy storage <ess> Saber/model/Temps/enhancedToWorkspace ==
  In1 : Inport  Port=1  LatchInput=off
  Terminator : Terminator
  wires:
  In1/1 -> Terminator/1

== system lib_energy_storage2/energy storage <ess> Saber/energy storage <ess> Saber/model/Temps/enhancedToWorkspace1 ==
  In1 : Inport  Port=1  LatchInput=off
  Terminator : Terminator
  wires:
  In1/1 -> Terminator/1

== system lib_energy_storage2/energy storage <ess> Saber/energy storage <ess> Saber/model/Thermal Power/enhancedToWorkspace ==
  In1 : Inport  Port=1  LatchInput=off
  Terminator : Terminator
  wires:
  In1/1 -> Terminator/1

== system lib_energy_storage2/energy storage <ess> Saber/energy storage <ess> Saber/model/Thermal Power/enhancedToWorkspace1 ==
  In1 : Inport  Port=1  LatchInput=off
  Terminator : Terminator
  wires:
  In1/1 -> Terminator/1

== system lib_energy_storage2/energy storage <ess> Saber/energy storage <ess> Saber/model/Time Dependent Power Request/Enabled Subsystem1 ==
  In1 : Inport  Port=1  LatchInput=off
  Enable : EnablePort
  Out1 : Outport  Port=1
  wires:
  In1/1 -> Out1/1

== system lib_energy_storage2/energy storage <ess> Saber/energy storage <ess> Saber/model/Voltages/enhancedToWorkspace ==
  In1 : Inport  Port=1  LatchInput=off
  Terminator : Terminator
  wires:
  In1/1 -> Terminator/1

== system lib_energy_storage2/energy storage <ess> Saber/energy storage <ess> Saber/model/Voltages/enhancedToWorkspace1 ==
  In1 : Inport  Port=1  LatchInput=off
  Terminator : Terminator
  wires:
  In1/1 -> Terminator/1

== system lib_energy_storage2/energy storage <ess> fundamental model/energy storage <ess> fundamental model/model/ess tmp/Block NOTES ==
  note: This block models the thermal behavior of a battery module with active air cooling.
      | The module is modeled as a single lumped thermal mass.
      | The fan is on whenever the battery temp is > the set temp.

== system lib_energy_storage2/energy storage <ess> fundamental model/energy storage <ess> fundamental model/model/ess tmp/Tair,ave ==
  Qess_case : Inport  Port=1  LatchInput=off
  Enable : EnablePort  StatesWhenEnabling=reset
  Block NOTES : Subsystem
      settings: RTWFcnNameOpts=Auto  RTWFileNameOpts=Auto
      mask Display: disp('Block\nNOTES')
  Tamb-(Q/mcp)/2 : Fcn  Expr=amb_tmp - (u(1)/(ess_mod_airflow*air_cp))/2
  do ex calcs?1 : Constant  Value=ess_th_res_on
  Tair_ave : Outport  Port=1  OutputWhenDisabled=reset  InitialOutput=amb_tmp
  Th Res : Outport  Port=2  OutputWhenDisabled=reset  InitialOutput=ess_th_res_off
  wires:
  do ex calcs?1/1 -> Th Res/1
  Qess_case/1 -> Tamb-(Q/mcp)/2/1
  Tamb-(Q/mcp)/2/1 -> Tair_ave/1

== system lib_energy_storage2/energy storage <ess> optima fundamental model/energy storage <ess> optima fundamental model/model/ess tmp/Block NOTES ==
  note: This block models the thermal behavior of a battery module with active air cooling.
      | The module is modeled as a single lumped thermal mass.
      | The fan is on whenever the battery temp is > the set temp.

== system lib_energy_storage2/energy storage <ess> optima fundamental model/energy storage <ess> optima fundamental model/model/ess tmp/Tair,ave ==
  Qess_case : Inport  Port=1  LatchInput=off
  Enable : EnablePort  StatesWhenEnabling=reset
  Block NOTES : Subsystem
      settings: RTWFcnNameOpts=Auto  RTWFileNameOpts=Auto
      mask Display: disp('Block\nNOTES')
  Tamb-(Q/mcp)/2 : Fcn  Expr=amb_tmp - (u(1)/(ess_mod_airflow*air_cp))/2
  do ex calcs?1 : Constant  Value=ess_th_res_on
  Tair_ave : Outport  Port=1  OutputWhenDisabled=reset  InitialOutput=amb_tmp
  Th Res : Outport  Port=2  OutputWhenDisabled=reset  InitialOutput=ess_th_res_off
  wires:
  do ex calcs?1/1 -> Th Res/1
  Qess_case/1 -> Tamb-(Q/mcp)/2/1
  Tamb-(Q/mcp)/2/1 -> Tair_ave/1

== system lib_energy_storage2/Ultracapacitor  System/Ultracapacitor  System/model/Calc Iout/limit power/Limits ==
  current req : Inport  Port=1  LatchInput=off
  current bat limited : Inport  Port=2  LatchInput=off
  V used : Inport  Port=3  LatchInput=off
  V mc_min_volts : Inport  Port=4  LatchInput=off
  V battery (.5Voc) : Inport  Port=5  LatchInput=off
  V ess_min_volts : Inport  Port=6  LatchInput=off
  Relational Operator1 : RelationalOperator  Operator===
  Relational Operator3 : RelationalOperator  Operator===
  Relational Operator4 : RelationalOperator  Operator===
  Relational Operator5 : RelationalOperator  Operator=<=
  limited by battery : Logic  Operator=AND  Inputs=2
  limited by battery min V : Logic  Operator=AND  Inputs=2
  limited by motor controller : Logic  Operator=AND  Inputs=2
  tag scope: ess_minV_limited=scoped, ess_pwr_limited=scoped, mc_voltage_limited=scoped
  wires:
  current bat limited/1 -> Relational Operator1/2
  V mc_min_volts/1 -> Relational Operator3/2
  V used/1 -> Relational Operator3/1, Relational Operator4/1, Relational Operator5/1
  V battery (.5Voc)/1 -> Relational Operator4/2
  V ess_min_volts/1 -> Relational Operator5/2
  limited by motor controller/1 -> [mc_voltage_limited]
  limited by battery/1 -> [ess_pwr_limited]
  limited by battery min V/1 -> [ess_minV_limited]
  Relational Operator3/1 -> limited by motor controller/2
  Relational Operator1/1 -> limited by motor controller/1, limited by battery/1, limited by battery min V/1
  Relational Operator4/1 -> limited by battery/2
  Relational Operator5/1 -> limited by battery min V/2
  current req/1 -> Relational Operator1/1

== system lib_energy_storage2/Ultracapacitor  System/Ultracapacitor  System/model/ess tmp/Tair,ave/Block NOTES ==
  note: This block determins the average temperature of the cooling air over the module.

== system lib_energy_storage2/energy storage <ess>/energy storage <ess>/Model/ess tmp/Tair,ave/Block NOTES ==
  note: This block determins the average temperature of the cooling air over the module.

== system lib_energy_storage2/energy storage <ess> RC/energy storage <ess> RC/model/Thermal Model of Battery/Tair,ave/Block NOTES ==
  note: This block determins the average temperature of the cooling air over the module.

== system lib_energy_storage2/energy storage <ess> nnet/energy storage <ess> nnet/model/NNet/Neural Network/Layer 1 ==
  "p{1}" : Inport  Port=1  LatchInput=off  PortDimensions=2
  Delays 1 : Subsystem
      settings: RTWFcnNameOpts=Auto  RTWFileNameOpts=Auto
      mask Display: disp('TDL')
  "IW{1,1}" : Subsystem
      settings: RTWFcnNameOpts=Auto  RTWFileNameOpts=Auto
      mask Display: disp('weight')
  "b{1}" : Constant  Value=[-6.0348629999999996;2.0410720000000002;2.002373]
      mask Display: disp('bias')
  logsig : Subsystem
      settings: RTWFcnNameOpts=Auto  RTWFileNameOpts=Auto
      mask Display: plot([-1 1],[0 0],[-1 -.9 -.8 -.7 -.6 -.5 -.4 -.3 -.2 -.1 0 .1 .2 .3 .4 .5 .6 .7 .8 .9 1],1./(1+exp(-8*[-1 -.9 -.8 -.7 -.6 -.5 -.4 -.3 -.2 -.1 0 .1 .2 .3 .4 .5 .6 .7 .8 .9 1]))+.01)
  netsum : Sum  Inputs=2  SaturateOnIntegerOverflow=on
      mask Display: disp('+')
  "a{1}" : Outport  Port=1  InitialOutput=[0;0;0]
  wires:
  logsig/1(a) -> "a{1}"/1
  netsum/1 -> logsig/1(n)
  "b{1}"/1 -> netsum/2
  "IW{1,1}"/1("iz{1,1}") -> netsum/1
  Delays 1/1("pd{1,1}") -> "IW{1,1}"/1("pd{1,1}")
  "p{1}"/1 -> Delays 1/1("p{1}")

== system lib_energy_storage2/energy storage <ess> nnet/energy storage <ess> nnet/model/NNet/Neural Network/Layer 2 ==
  "a{1} " : Inport  Port=1  LatchInput=off  PortDimensions=3
  Delays 1 : Subsystem
      settings: RTWFcnNameOpts=Auto  RTWFileNameOpts=Auto
      mask Display: disp('TDL')
  "LW{2,1}" : Subsystem
      settings: RTWFcnNameOpts=Auto  RTWFileNameOpts=Auto
      mask Display: disp('weight')
  "b{2}" : Constant  Value=[3.0652170000000001;-2.2814760000000001]
      mask Display: disp('bias')
  logsig : Subsystem
      settings: RTWFcnNameOpts=Auto  RTWFileNameOpts=Auto
      mask Display: plot([-1 1],[0 0],[-1 -.9 -.8 -.7 -.6 -.5 -.4 -.3 -.2 -.1 0 .1 .2 .3 .4 .5 .6 .7 .8 .9 1],1./(1+exp(-8*[-1 -.9 -.8 -.7 -.6 -.5 -.4 -.3 -.2 -.1 0 .1 .2 .3 .4 .5 .6 .7 .8 .9 1]))+.01)
  netsum : Sum  Inputs=2  SaturateOnIntegerOverflow=on
      mask Display: disp('+')
  "a{2}" : Outport  Port=1  InitialOutput=[0;0]
  wires:
  logsig/1(a) -> "a{2}"/1
  netsum/1 -> logsig/1(n)
  "b{2}"/1 -> netsum/2
  "LW{2,1}"/1("lz{2,1}") -> netsum/1
  Delays 1/1("pd{2,1}") -> "LW{2,1}"/1("ad{2,1}")
  "a{1} "/1 -> Delays 1/1("p{2}")

== system lib_energy_storage2/energy storage <ess> fundamental model/energy storage <ess> fundamental model/model/ess tmp/Tair,ave/Block NOTES ==
  note: This block determins the average temperature of the cooling air over the module.

== system lib_energy_storage2/energy storage <ess> optima fundamental model/energy storage <ess> optima fundamental model/model/ess tmp/Tair,ave/Block NOTES ==
  note: This block determins the average temperature of the cooling air over the module.

== system lib_energy_storage2/energy storage <ess> nnet/energy storage <ess> nnet/model/NNet/Neural Network/Layer 1/Delays 1 ==
  "p{1}" : Inport  Orientation=down  Port=1  LatchInput=off  PortDimensions=2
  mux : Mux  Inputs=1
      settings: DisplayOption=none
  "pd{1,1}" : Outport  Port=1  InitialOutput=0
  wires:
  mux/1 -> "pd{1,1}"/1
  "p{1}"/1 -> mux/1

== system lib_energy_storage2/energy storage <ess> nnet/energy storage <ess> nnet/model/NNet/Neural Network/Layer 1/IW{1,1} ==
  "pd{1,1}" : Inport  Port=1  LatchInput=off  PortDimensions=2
  "IW{1,1}(1,:)'" : Constant  Value=[-4.5598890000000001;5.793647]
      mask Display: disp('weights')
  "IW{1,1}(2,:)'" : Constant  Value=[-2.8283469999999999;1.417519]
      mask Display: disp('weights')
  "IW{1,1}(3,:)'" : Constant  Value=[-2.3043559999999998;-1.4467429999999999]
      mask Display: disp('weights')
  Mux : Mux  Inputs=3
      settings: DisplayOption=none
  dotprod1 : Subsystem
      settings: RTWFcnNameOpts=Auto  RTWFileNameOpts=Auto
  dotprod2 : Subsystem
      settings: RTWFcnNameOpts=Auto  RTWFileNameOpts=Auto
  dotprod3 : Subsystem
      settings: RTWFcnNameOpts=Auto  RTWFileNameOpts=Auto
  "iz{1,1}" : Outport  Port=1  InitialOutput=0
  wires:
  Mux/1 -> "iz{1,1}"/1
  dotprod3/1(z) -> Mux/3
  "IW{1,1}(3,:)'"/1 -> dotprod3/1(w)
  dotprod2/1(z) -> Mux/2
  "pd{1,1}"/1 -> dotprod3/2(p), dotprod2/2(p), dotprod1/2(p)
  "IW{1,1}(2,:)'"/1 -> dotprod2/1(w)
  dotprod1/1(z) -> Mux/1
  "IW{1,1}(1,:)'"/1 -> dotprod1/1(w)

== system lib_energy_storage2/energy storage <ess> nnet/energy storage <ess> nnet/model/NNet/Neural Network/Layer 1/logsig ==
  n : Inport  Port=1  LatchInput=off
  Exp : ElementaryMath  Operator=exp
  Gain : Gain  Gain=-1  Multiplication=Element-wise(K.*u)  SaturateOnIntegerOverflow=on
  Reciprocal : ElementaryMath  Operator=reciprocal
  Sum : Sum  Inputs=++  SaturateOnIntegerOverflow=on
  one : Constant  Value=1
  a : Outport  Port=1  InitialOutput=0
  wires:
  n/1 -> Gain/1
  Gain/1 -> Exp/1
  Exp/1 -> Sum/1
  one/1 -> Sum/2
  Sum/1 -> Reciprocal/1
  Reciprocal/1 -> a/1

== system lib_energy_storage2/energy storage <ess> nnet/energy storage <ess> nnet/model/NNet/Neural Network/Layer 2/Delays 1 ==
  "p{2}" : Inport  Orientation=down  Port=1  LatchInput=off  PortDimensions=3
  mux : Mux  Inputs=1
      settings: DisplayOption=none
  "pd{2,1}" : Outport  Port=1  InitialOutput=0
  wires:
  mux/1 -> "pd{2,1}"/1
  "p{2}"/1 -> mux/1
